simulink model "rotpentemplate_with_deadzone_comp"  (R2020b)
settings: Solver=ode45  StartTime=0.0  StopTime=10  RelTol=1e-3  EnableMultiTasking=on
values from neighbouring files (symbols this model uses):
  b1 = 5.33518    [Linearization.m]    (also in MainScript_PID.m; calib_up_up.m; tune_parameters.m = 4.8; tune_parameters_cl.m)
  b2 = 4e-05    [Linearization.m]    (also in MainScript_PID.m; calib_up_up.m; tune_parameters.m = 5e-05; tune_parameters_cl.m = 3.7644e-05)
  g01 = mean_data(2)    [MainScript_PID.m]    (also in calib_up_up.m)
  g02 = mean_data(3)    [MainScript_PID.m]    (also in calib_up_up.m)
  g1 = (m1*c1+m2*l1)*g    (= 0.097031577204)    [Linearization.m]    (also in calib_up_up.m)
  g11 = (mean_data(2)-mean_data(1))/pi    [MainScript_PID.m]    (also in calib_up_up.m)
  g12 = (mean_data(3)-mean_data(4))/pi    [MainScript_PID.m]    (also in calib_up_up.m)
  g2 = m2*c2*g    (= 0.0604103724)    [Linearization.m]    (also in calib_up_up.m)
  h = 0.01    [MainScript_PID.m]    (also in calib_up_up.m = 0.005)
  km = 39.2954    [Linearization.m]    (also in MainScript_PID.m = 42.2954; calib_up_up.m; tune_parameters.m = 50; tune_parameters_cl.m)
  P1 = m1*c1^2 + m2*l1^2 + I1    (= 0.0114878306295)    [Linearization.m]    (also in calib_up_up.m)
  P2 = m2*c2^2 + I2    (= 0.0005310628)    [Linearization.m]    (also in calib_up_up.m)
  P3 = m2*l1*c2    (= 0.000552376188)    [Linearization.m]    (also in calib_up_up.m)
  te = 0.01    [Linearization.m]    (also in MainScript_PID.m = 0.008; calib_up_up.m; tune_parameters.m = 0.03; tune_parameters_cl.m = 0.00258)
  theta0 = [-pi;3*pi/4]    [Compute_whitebox.m]    (also in MainScript_PID.m = [-pi;     pi/4]; calib_up_up.m = [0;-pi]; tune_parameters.m = [-pi;10*pi/12]; tune_parameters_cl.m = [-pi;-pi])
  thetadot0 = [0;0]    [MainScript_PID.m]    (also in calib_up_up.m; tune_parameters.m; tune_parameters_cl.m; tune_parameters_theta1.m)
undefined symbols (not defined in the file or in its folder): adingain, adinoffs, daoutgain, daoutoffs
libraries: dspsigops x4
settings Model: Creator=rbabuska  LastModifiedBy=cmatteo
settings DataIOCC: LimitDataPoints=on  SaveFormat=Array  ReturnWorkspaceOutputs=off  SignalLoggingName=sigsOut
settings OptimizationCC: BooleanDataType=off  ExpressionDepthLimit=2147483647  InitFltsAndDblsToZero=on  LifeSpan=inf
settings DebuggingCC: SaveWithParameterizedLinksMsg=none  SignalResolutionControl=TryResolveAllWithWarning  MultiTaskDSMMsg=warning  MultiTaskCondExecSysMsg=none  AllowSymbolicDim=off  StateNameClashWarn=warning  SFUnexpectedBacktrackingDiag=warning  SFNoUnconditionalDefaultTransitionDiag=warning  SFExecutionAtInitializationDiag=none  ArithmeticOperatorsInVariantConditions=warning
settings HardwareCC: ProdBitPerPointer=32  ProdBitPerSizeT=32  ProdBitPerPtrDiffT=32  ProdLargestAtomicFloat=None  ProdIntDivRoundTo=Undefined  ProdEndianess=Unspecified  ProdWordSize=32  ProdHWDeviceType=32-bit Generic  TargetUnknown=on
settings ModelReferenceCC: PropagateSignalLabelsOutOfModel=off
settings SFSimCC: SimUseLocalCustomCode=off  CustomCodeUndefinedFunction=UseInterfaceOnly
settings RTWCC: RTWUseLocalCustomCode=off
settings CodeAppCC: StateflowObjectComments=on
settings GRTTargetCC: TargetFcnLib=ansi_tfl_tmw.mat  TargetLangStandard=C89/C90 (ANSI)  CombineOutputUpdateFcns=off  GRTInterface=on
settings ConfigComp: CovMetricSettings=dw  CovSaveCumulativeToWorkspaceVar=on  CovSaveSingleToWorkspaceVar=on  CovExternalEMLEnable=off

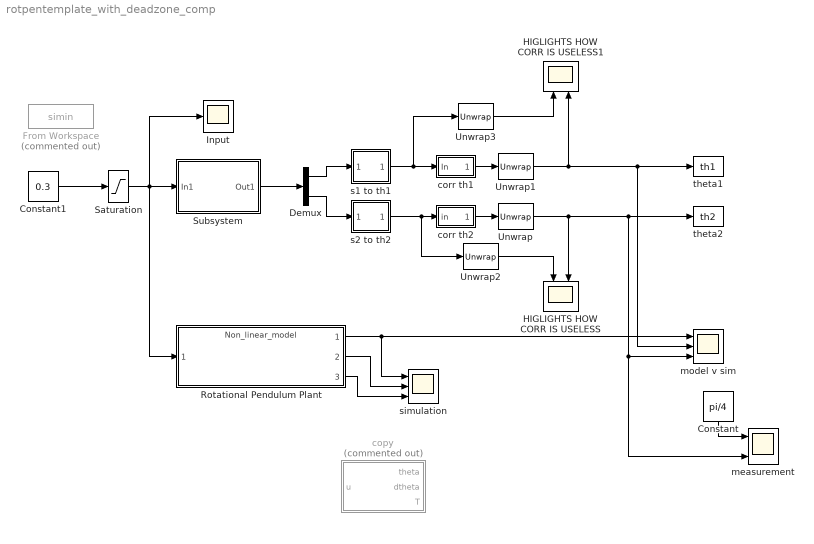
== system rotpentemplate_with_deadzone_comp ==
  Constant : Constant  Value=pi/4
  Constant1 : Constant  Value=0.3
  Demux : Demux  Outputs=2
  From Workspace : FromWorkspace  Commented=on  VariableName=simin
  HIGLIGHTS HOW CORR IS USELESS : Scope  NumInputPorts=2
  HIGLIGHTS HOW CORR IS USELESS1 : Scope  NumInputPorts=2
  Input : Scope
  Rotational Pendulum Plant : ModelReference  ModelNameDialog=Non_linear_model.slx  SimulationMode=Normal  ModelReferenceVersion=3.13
  Saturation : Saturate  UpperLimit=1  LowerLimit=-1
  Subsystem : Subsystem
      mask Display: disp('Rotational\nPendulum')
  Unwrap{,1..3} (4 alike) : dspsigops/Unwrap  tol=pi  InputProcessing=Columns as channels (frame based)  running=off
  copy : Subsystem  Commented=on
  corr th1 : Subsystem
  corr th2 : Subsystem
  measurement : Scope  NumInputPorts=2
  model v sim : Scope  NumInputPorts=3
  s1 to th1 : Subsystem
  s2 to th2 : Subsystem
  simulation : Scope  NumInputPorts=3
  theta1 : ToWorkspace  VariableName=th1  SaveFormat=Timeseries  SampleTime=-1
  theta2 : ToWorkspace  VariableName=th2  SaveFormat=Timeseries  SampleTime=-1
  wires:
  Saturation/1 -> Rotational Pendulum Plant/1, Input/1, Subsystem/1(In1)
  Subsystem/1(Out1) -> Demux/1
  Demux/1 -> s1 to th1/1(v1)
  Demux/2 -> s2 to th2/1(v2)
  Constant1/1 -> Saturation/1
  s2 to th2/1(th2) -> Unwrap2/1, corr th2/1(in)
  s1 to th1/1(th1) -> corr th1/1(In), Unwrap3/1
  Unwrap/1 -> HIGLIGHTS HOW CORR IS USELESS/2, measurement/2, model v sim/3, theta2/1
  corr th2/1(corr) -> Unwrap/1
  corr th1/1(Corr) -> Unwrap1/1
  Unwrap1/1 -> model v sim/2, theta1/1, HIGLIGHTS HOW CORR IS USELESS1/2
  Constant/1 -> measurement/1
  Rotational Pendulum Plant/1 -> simulation/1, model v sim/1
  Rotational Pendulum Plant/2 -> simulation/2
  Rotational Pendulum Plant/3 -> simulation/3
  Unwrap2/1 -> HIGLIGHTS HOW CORR IS USELESS/1
  Unwrap3/1 -> HIGLIGHTS HOW CORR IS USELESS1/1

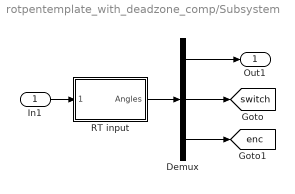
== system rotpentemplate_with_deadzone_comp/Subsystem ==
  In1 : Inport
  Demux : Demux  Outputs=[2 4 1]
  RT input : Subsystem  mask{Ts=h, channels=[6 7]}
      mask prompts: Ts "Sample time [s]:"; channels "Channels to read (e.g., [6 7])"
      mask init:
      | hwinit;
      | 
      | % initialize FPGA
      | fugihandle = fugiboard('Open', 'Pendulum1');
      | fugihandle.WatchdogTimeout = 0.5;
      | fugiboard('SetParams', fugihandle);
      | fugiboard('Write', fugihandle, 0, 0, 0, 0);  % dummy write to sync interface board
      | fugiboard('Write', fugihandle, 5, 1, 0, 0);  % reset position, activate relay
      | data = fugiboard('Read', fugihandle);        % get version info from FPGA
      | % model = bitshift(data(1), -5); 
      | % version = bitand(data(1), 31);
      | % disp(sprintf('FPGA setup %d, version %d', model, version)); % for the B&P it should say 1 1, or else there is a problem
      | fugiboard('Write', fugihandle, 0, 1, 0, 0);  % end reset
      | pause(0.1);                         % give relay some time to respond
      mask Display: disp('Rotational\nPendulum')
  Out1 : Outport
  tag scope: enc=global, switch=global
  wires:
  RT input/1(Angles) -> Demux/1
  Demux/1 -> Out1/1
  Demux/2 -> [switch]
  Demux/3 -> [enc]
  In1/1 -> RT input/1(Motors)

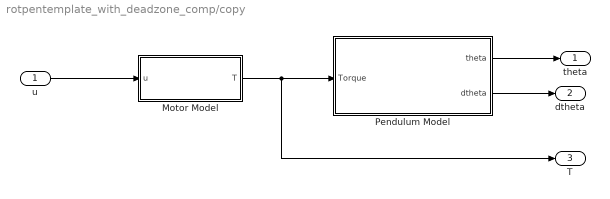
== system rotpentemplate_with_deadzone_comp/copy ==
  u : Inport
  "Motor Model " : Subsystem
  Pendulum Model : Subsystem
  theta : Outport
  dtheta : Outport  Port=2
  T : Outport  Port=3
  wires:
  Pendulum Model/1(theta) -> theta/1
  "Motor Model "/1(T) -> T/1, Pendulum Model/1(Torque)
  u/1 -> "Motor Model "/1(u)
  Pendulum Model/2(dtheta) -> dtheta/1

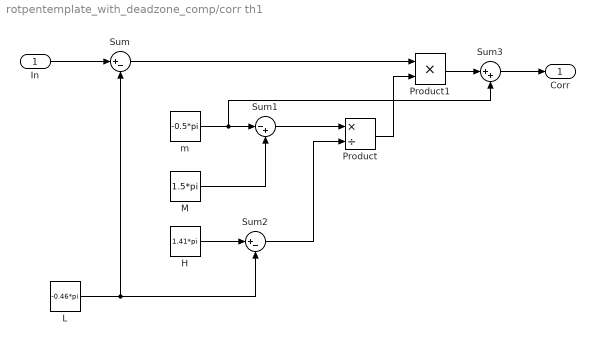
== system rotpentemplate_with_deadzone_comp/corr th1 ==
  In : Inport
  H : Constant  Value=1.41*pi
  L : Constant  Value=-0.46*pi
  M : Constant  Value=1.5*pi
  Product : Product  Inputs=*/
  Product1 : Product
  Sum : Sum  Inputs=|+-
  Sum1 : Sum  Inputs=|-+
  Sum2 : Sum  Inputs=|+-
  Sum3 : Sum  Inputs=|++
  m : Constant  Value=-0.5*pi
  Corr : Outport
  wires:
  L/1 -> Sum2/2, Sum/2
  M/1 -> Sum1/2
  Sum1/1 -> Product/1
  m/1 -> Sum3/2, Sum1/1
  Product1/1 -> Sum3/1
  Product/1 -> Product1/2
  Sum/1 -> Product1/1
  Sum2/1 -> Product/2
  Sum3/1 -> Corr/1
  H/1 -> Sum2/1
  In/1 -> Sum/1

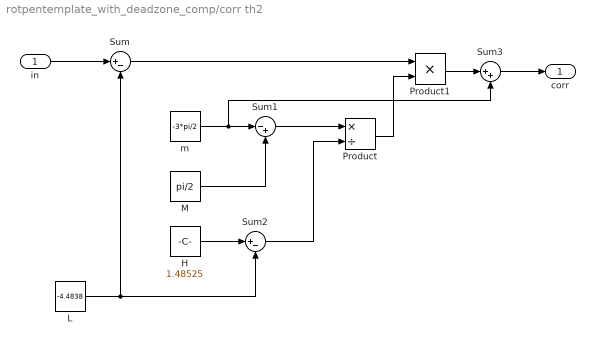
== system rotpentemplate_with_deadzone_comp/corr th2 ==
  in : Inport
  H : Constant  Value=1.48525
  L : Constant  Value=-4.4838
  M : Constant  Value=pi/2
  Product : Product  Inputs=*/
  Product1 : Product
  Sum : Sum  Inputs=|+-
  Sum1 : Sum  Inputs=|-+
  Sum2 : Sum  Inputs=|+-
  Sum3 : Sum  Inputs=|++
  m : Constant  Value=-3*pi/2
  corr : Outport
  wires:
  in/1 -> Sum/1
  M/1 -> Sum1/2
  m/1 -> Sum3/2, Sum1/1
  H/1 -> Sum2/1
  L/1 -> Sum2/2, Sum/2
  Sum1/1 -> Product/1
  Sum2/1 -> Product/2
  Sum/1 -> Product1/1
  Product/1 -> Product1/2
  Product1/1 -> Sum3/1
  Sum3/1 -> corr/1

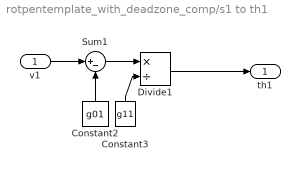
== system rotpentemplate_with_deadzone_comp/s1 to th1 ==
  v1 : Inport
  Constant2 : Constant  Value=g01
  Constant3 : Constant  Value=g11
  Divide1 : Product  Inputs=*/
  Sum1 : Sum  Inputs=|+-
  th1 : Outport
  wires:
  Constant2/1 -> Sum1/2
  Constant3/1 -> Divide1/2
  Divide1/1 -> th1/1
  Sum1/1 -> Divide1/1
  v1/1 -> Sum1/1

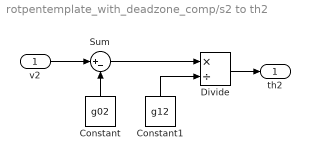
== system rotpentemplate_with_deadzone_comp/s2 to th2 ==
  v2 : Inport
  Constant : Constant  Value=g02
  Constant1 : Constant  Value=g12
  Divide : Product  Inputs=*/
  Sum : Sum  Inputs=|+-
  th2 : Outport
  wires:
  Constant1/1 -> Divide/2
  Divide/1 -> th2/1
  Constant/1 -> Sum/2
  Sum/1 -> Divide/1
  v2/1 -> Sum/1

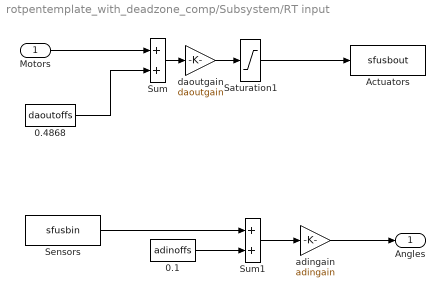
== system rotpentemplate_with_deadzone_comp/Subsystem/RT input ==
  Motors : Inport
  0.1 : Constant  Value=adinoffs
  0.4868 : Constant  Value=daoutoffs
  Actuators : S-Function  FunctionName=sfusbout  Parameters=Ts, fugihandle  SFunctionDeploymentMode=off  EnableBusSupport=off
  Saturation1 : Saturate  UpperLimit=10  LowerLimit=-10
  Sensors : S-Function  FunctionName=sfusbin  Parameters=Ts, fugihandle, channels  SFunctionDeploymentMode=off  EnableBusSupport=off
  Sum : Sum  InputSameDT=on  SaturateOnIntegerOverflow=on  OutDataTypeStr=Inherit: Same as first input
  Sum1 : Sum  InputSameDT=on  SaturateOnIntegerOverflow=on  OutDataTypeStr=Inherit: Same as first input
  adingain : Gain  Gain=adingain  SaturateOnIntegerOverflow=on  OutDataTypeStr=Inherit: Same as input  ParamDataTypeStr=Inherit: Same as input
  daoutgain : Gain  Gain=daoutgain  SaturateOnIntegerOverflow=on  OutDataTypeStr=Inherit: Same as input  ParamDataTypeStr=Inherit: Same as input
  Angles : Outport
  wires:
  Sum/1 -> daoutgain/1
  0.4868/1 -> Sum/2
  Motors/1 -> Sum/1
  Sum1/1 -> adingain/1
  0.1/1 -> Sum1/2
  adingain/1 -> Angles/1
  Saturation1/1 -> Actuators/1
  daoutgain/1 -> Saturation1/1
  Sensors/1 -> Sum1/1

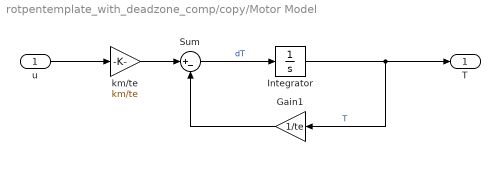
== system rotpentemplate_with_deadzone_comp/copy/Motor Model  ==
  u : Inport
  Gain1 : Gain  Gain=1/te
  Integrator : Integrator
  Sum : Sum  Inputs=|+-
  "km/te " : Gain  Gain=km/te
  T : Outport
  wires:
  "km/te "/1 -> Sum/1
  u/1 -> "km/te "/1
  Integrator/1 -> T/1, Gain1/1  "T"
  Sum/1 -> Integrator/1  "dT"
  Gain1/1 -> Sum/2

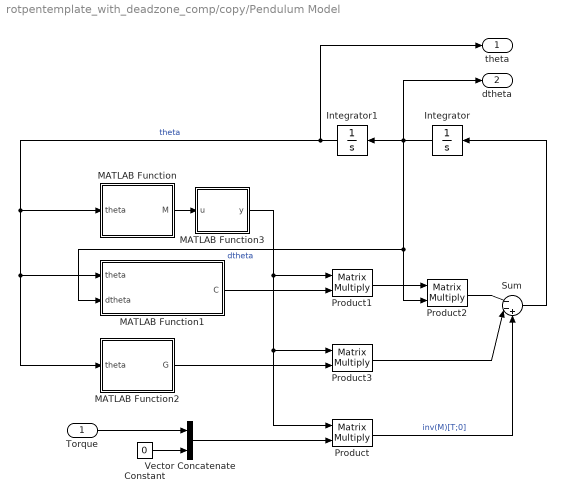
== system rotpentemplate_with_deadzone_comp/copy/Pendulum Model ==
  Torque : Inport
  Constant : Constant  Value=0
  Integrator : Integrator  InitialCondition=[thetadot0(1);thetadot0(2)]
  Integrator1 : Integrator  InitialCondition=[theta0(1);theta0(2)]
  MATLAB Function : MATLAB Function  TreatAsAtomicUnit=on
  MATLAB Function1 : MATLAB Function  TreatAsAtomicUnit=on
  MATLAB Function2 : MATLAB Function  TreatAsAtomicUnit=on
  MATLAB Function3 : MATLAB Function  TreatAsAtomicUnit=on
  Product{,1..3} (4 alike) : Product  Multiplication=Matrix(*)
  Sum : Sum  Inputs=|--+
  Vector Concatenate : Concatenate
  theta : Outport
  dtheta : Outport  Port=2
  wires:
  Product/1 -> Sum/3  "inv(M)[T;0]"
  MATLAB Function3/1(y) -> Product3/1, Product/1, Product1/1
  Product1/1 -> Product2/1
  MATLAB Function/1(M) -> MATLAB Function3/1(u)
  Integrator/1 -> dtheta/1, MATLAB Function1/2(dtheta), Product2/2, Integrator1/1  "dtheta"
  Product3/1 -> Sum/2
  Integrator1/1 -> theta/1, MATLAB Function/1(theta), MATLAB Function2/1(theta), MATLAB Function1/1(theta)  "theta"
  Sum/1 -> Integrator/1
  MATLAB Function2/1(G) -> Product3/2
  MATLAB Function1/1(C) -> Product1/2
  Product2/1 -> Sum/1
  Torque/1 -> Vector Concatenate/1
  Constant/1 -> Vector Concatenate/2
  Vector Concatenate/1 -> Product/2

== matlab function rotpentemplate_with_deadzone_comp/copy/Pendulum Model/MATLAB Function1 ==
  data: theta input; C output; dtheta input; b1 parameter; P3 parameter; b2 parameter
function C = C_matrix(theta, dtheta,b1,P3, b2)
C = [b1-P3*dtheta(2)*sin(theta(2))  -P3*(dtheta(1)+dtheta(2))*sin(theta(2));
     P3*dtheta(1)*sin(theta(2))     b2];

== matlab function rotpentemplate_with_deadzone_comp/copy/Pendulum Model/MATLAB Function ==
  data: theta input size=2; M output; P1 parameter; P3 parameter; P2 parameter
function M = M_matrix(theta,P1, P3, P2)
    M = [P1+P2+2*P3*cos(theta(2)) P2+P3*cos(theta(2));
         P2+P3*cos(theta(2))      P2];

== matlab function rotpentemplate_with_deadzone_comp/copy/Pendulum Model/MATLAB Function2 ==
  data: theta input; G output; g2 parameter; g1 parameter
function G = G_matrix(theta,g2,g1)
G = [-g1*sin(theta(1))-g2*sin(theta(1)+theta(2));
     -g2*sin(theta(1)+theta(2))];

== matlab function rotpentemplate_with_deadzone_comp/copy/Pendulum Model/MATLAB Function3 ==
  data: u input; y output
function y = inverse(u)
y = inv(u);
